simulink model "case1_2"  (R2022b)
settings: Solver=VariableStepAuto  StartTime=0.0  StopTime=40.0  RelTol=1e-3
values from neighbouring files (symbols this model uses):
  K1_new = 26.7    [main.m]
  Kd_new = 0.0435    [main.m]
  Ke_new = 1.237    [main.m]
  wmax = 150    [main.m]
libraries: fuzblock x1
settings Model: Creator=karam  LastModifiedBy=kmpouzio
settings SolverCC: AlgebraicLoopSolver=TrustRegion
settings DebuggingCC: UnconnectedInputMsg=warning  UnconnectedOutputMsg=warning  UnconnectedLineMsg=warning  SFMachineParentedDataDiag=warning
settings ModelReferenceCC: EnableRefExpFcnMdlSchedulingChecks=on

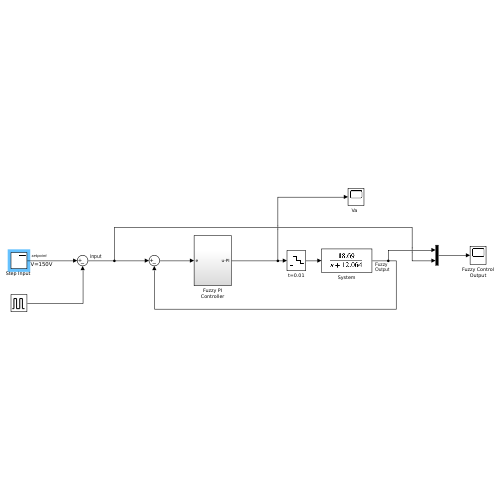
[thumbnail: Simulink's stored preview of the top-level diagram]
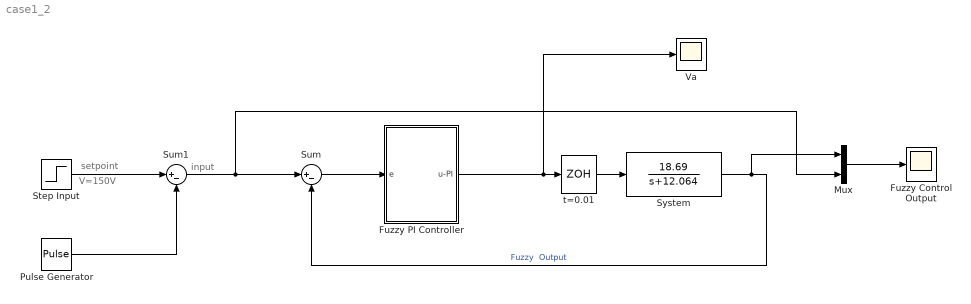
== system case1_2 ==
  note: input
  note: V=150V
  note: setpoint
  Fuzzy Control Output : Scope
  Fuzzy PI Controller : Subsystem
  Mux : Mux  Inputs=2
  Pulse Generator : DiscretePulseGenerator  PulseType=Time based  Amplitude=50  Period=20  PulseWidth=50  PhaseDelay=-90
  "Step Input " : Step  Time=0  After=wmax  SampleTime=0.1
  Sum : Sum  Inputs=|+-  SaturateOnIntegerOverflow=on
  Sum1 : Sum  Inputs=|+-  SaturateOnIntegerOverflow=on
  System : TransferFcn  Numerator=[18.69]  Denominator=[1 12.064]
  "Va  " : Scope
  t=0.01 : ZeroOrderHold  SampleTime=0.01
  wires:
  t=0.01/1 -> System/1
  Fuzzy PI Controller/1(u-PI) -> "Va  "/1, t=0.01/1
  System/1 -> Sum/2, Mux/1  "Fuzzy  Output"
  Sum/1 -> Fuzzy PI Controller/1(e)
  Mux/1 -> Fuzzy Control Output/1
  "Step Input "/1 -> Sum1/1
  Pulse Generator/1 -> Sum1/2
  Sum1/1 -> Mux/2, Sum/1

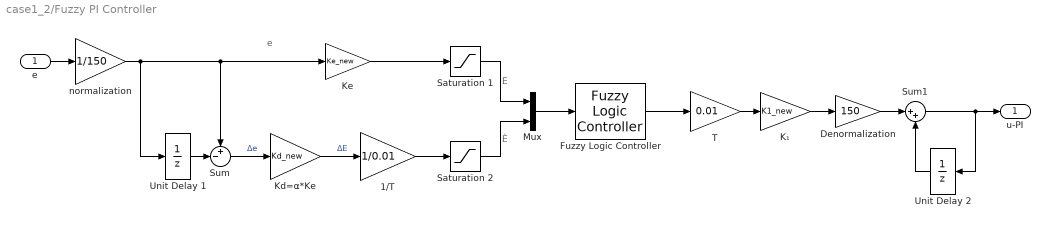
== system case1_2/Fuzzy PI Controller ==
  note: e
  note: E
  note: Ė
  e : Inport
  1/T : Gain  Gain=1/0.01  SaturateOnIntegerOverflow=on  OutDataTypeStr=Inherit: Same as input  ParamDataTypeStr=Inherit: Same as input
  Denormalization : Gain  Gain=150  SaturateOnIntegerOverflow=on  OutDataTypeStr=Inherit: Same as input  ParamDataTypeStr=Inherit: Same as input
  Fuzzy Logic Controller : fuzblock/Fuzzy Logic  Controller  FIS='FLC07.fis'  OutputSampleNumber=101  DataType=double  FuzzifiedInputs=off  RuleFiringStrengths=off  RuleOutputs=off  AggregatedOutputs=off  SimulateUsing=Interpreted execution  OutOfRangeInputValueMessage=warning  NoRuleFiredMessage=warning  EmptyOutputFuzzySetMessage=warning
  Kd=α*Ke : Gain  Gain=Kd_new  SaturateOnIntegerOverflow=on  OutDataTypeStr=Inherit: Same as input  ParamDataTypeStr=Inherit: Same as input
  Ke : Gain  Gain=Ke_new  SaturateOnIntegerOverflow=on  OutDataTypeStr=Inherit: Same as input  ParamDataTypeStr=Inherit: Same as input
  K₁ : Gain  Gain=K1_new  SaturateOnIntegerOverflow=on  OutDataTypeStr=Inherit: Same as input  ParamDataTypeStr=Inherit: Same as input
  Mux : Mux  Inputs=2
  Saturation 1 : Saturate  UpperLimit=1  LowerLimit=-1
  Saturation 2 : Saturate  UpperLimit=1  LowerLimit=-1
  Sum : Sum  Inputs=+-|  SaturateOnIntegerOverflow=on
  Sum1 : Sum  Inputs=|++  SaturateOnIntegerOverflow=on
  T : Gain  Gain=0.01  SaturateOnIntegerOverflow=on  OutDataTypeStr=Inherit: Same as input  ParamDataTypeStr=Inherit: Same as input
  Unit Delay 1 : UnitDelay  SampleTime=0.01  HasFrameUpgradeWarning=on
  Unit Delay 2 : UnitDelay  SampleTime=0.01  HasFrameUpgradeWarning=on
  normalization : Gain  Gain=1/150  SaturateOnIntegerOverflow=on  OutDataTypeStr=Inherit: Same as input  ParamDataTypeStr=Inherit: Same as input
  u-PI : Outport  VectorParamsAs1DForOutWhenUnconnected=off
  wires:
  e/1 -> normalization/1
  normalization/1 -> Unit Delay 1/1, Ke/1, Sum/1
  Ke/1 -> Saturation 1/1
  Saturation 1/1 -> Mux/1
  T/1 -> K₁/1
  K₁/1 -> Denormalization/1
  Denormalization/1 -> Sum1/1
  Sum1/1 -> u-PI/1, Unit Delay 2/1
  Unit Delay 2/1 -> Sum1/2
  Unit Delay 1/1 -> Sum/2
  Sum/1 -> Kd=α*Ke/1  "Δe"
  Kd=α*Ke/1 -> 1/T/1  "ΔE"
  1/T/1 -> Saturation 2/1
  Saturation 2/1 -> Mux/2
  Mux/1 -> Fuzzy Logic Controller/1
  Fuzzy Logic Controller/1 -> T/1
